simulink model "bandpass_complex_PAM_channel"  (R2016b)
settings: Solver=ode45  StartTime=0.0  StopTime=1000  RelTol=1e-3  EnableMultiTasking=on
InitFcn:
  | close all;
  | bandpass_complex_PAM_channel_ini;
StopFcn:
  | figure(1),
  | n=1:min([1000 length(srx)]);
  | subplot(211),plot(n,real(srx(n)),'.');
  | title('Real(srx)');
  | subplot(212),plot(n,imag(srx(n)),'.');
  | title('Imag(srx)');
undefined symbols (not defined in the file or in its folder): j
libraries: commfilt2 x2, commnoisgen2 x1, commrandsrc2 x1, commdigbbndam3 x1, commsink2 x1, commutil2 x1, dspobslib x1
settings Model: Creator=erban  LastModifiedBy=erban
settings DataIOCC: LimitDataPoints=on  SaveFormat=Array  SignalLoggingSaveFormat=ModelDataLogs  SignalLoggingName=sigsOut
settings OptimizationCC: BooleanDataType=off
settings DebuggingCC: SaveWithParameterizedLinksMsg=none  UnderspecifiedInitializationDetection=Classic  MergeDetectMultiDrivingBlocksExec=none  SignalResolutionControl=TryResolveAllWithWarning  MultiTaskDSMMsg=warning  MultiTaskCondExecSysMsg=none
settings HardwareCC: ProdBitPerPointer=32  ProdBitPerSizeT=32  ProdBitPerPtrDiffT=32  ProdLargestAtomicFloat=None  ProdIntDivRoundTo=Undefined  ProdEndianess=Unspecified  ProdWordSize=32  ProdHWDeviceType=32-bit Generic  TargetUnknown=on
settings ModelReferenceCC: PropagateSignalLabelsOutOfModel=off
settings GRTTargetCC: TargetLangStandard=C89/C90 (ANSI)  CombineOutputUpdateFcns=off  GRTInterface=on
settings ConfigComp: CovMetricSettings=dw  CovHtmlReporting=on  CovSaveCumulativeToWorkspaceVar=on  CovSaveSingleToWorkspaceVar=on  CovExternalEMLEnable=off

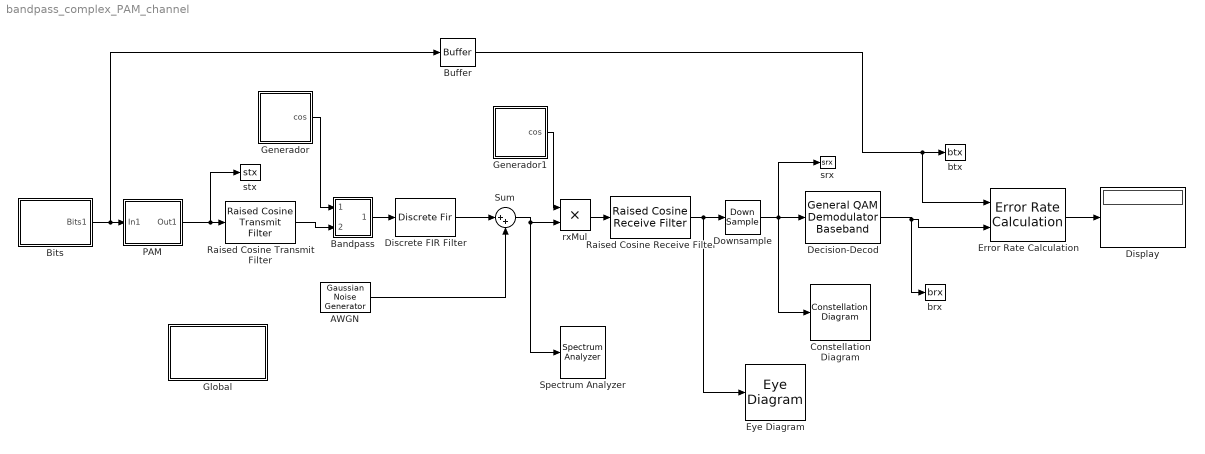
== system bandpass_complex_PAM_channel ==
  AWGN : commnoisgen2/Gaussian Noise Generator  m=0  d=1e-6  s=floor(60 * rand)+1  Ts=-1  frameBased=off  sampPerFrame=64  orient=off  outDataType=double
  Bandpass : Subsystem
      mask Display: disp('x Re{.}');
  Bits : Subsystem
      mask Display: disp('11001010');
  Buffer : Buffer  N=2  TreatMby1Signals=One channel  OutputFrames=off
  Constellation Diagram : ConstellationDiagram
  Decision-Decod : commdigbbndam3/General QAM Demodulator Baseband  SigCon=[1+j,-1+j,1-j,-1-j]  OutType=Bit  DecType=Hard decision  VarSource=Dialog  Variance=1  outDtypeBit=Inherit via internal rule  outDtype=Inherit via internal rule  roundingMode=Floor  overflowMode=Wrap  OvFlMode=off  OvFlModeLastStrValue=off  sigConstWordLen=16  sigConstDataTypeStr=Inherit: Same word length as input  sigConstLastDataTypeStr=Inherit: Same word length as input  accum1WordLen=32  accum1FracLen=30  prodInWordLen=32  prodInFracLen=30  prodInDataTypeStr=Inherit: Same as accumulator 1  prodInLastDataTypeStr=Inherit: Same as accumulator 1  prodOutWordLen=32  prodOutFracLen=30  accum2WordLen=32  accum2FracLen=30  accum3WordLen=32  accum3FracLen=30  nsiWordLen=32  nsiFracLen=30  nsiDataTypeStr=Inherit: Same as accumulator 3  nsiLastDataTypeStr=Inherit: Same as accumulator 3  invn0WordLen=16  invn0FracLen=8  invn0DataTypeStr=Inherit: Same word length as input  invn0LastDataTypeStr=Inherit: Same word length as input  outputWordLen=32  outputFracLen=30
  Discrete FIR Filter : DiscreteFir  Coefficients=1
  Display : Display
  Downsample : DownSample  N=128  RateOptions=Allow multirate processing
  Error Rate Calculation : commsink2/Error Rate Calculation  N=20  st_delay=50  cp_mode=Entire frame  subframe=[]  PMode=Port  WsName=ErrorVec  RsMode2=off  stop=off  numErr=100  maxBits=1e6
  Eye Diagram : EyeDiagram
  Generador : Subsystem  mask(SenCos){desfase=0, frec=1e4}
      mask prompts: frec "Frecuencia (Hz)"
      mask help: Saca un seno y un coseno de la frecuencia y la fase dadas.
      mask Display: disp('Complex \n exp(j.)');
  Generador1 : Subsystem  mask(SenCos){desfase=0, frec=10000}
      mask prompts: frec "Frecuencia (Hz)"
      mask help: Saca un seno y un coseno de la frecuencia y la fase dadas.
      mask Display: disp('Complex \n exp(-j.)');
  Global : Subsystem  mask{constellation=[1+j,-1+j,1-j,-1-j], Rb=1000, fc=1e4, NoiseVar=1e-6, channel=1, CFreqD=0, CPhasD=0, SPerD=0, SPhasD=0}
      mask prompts: fc "fc (Hz)"; channel "FIR channel"; CFreqD "Freq. Dev. (% fc)"; CPhasD "Phase Dev. (rad)"; SPerD "Symbol Period Dev. (% T)"; SPhasD "Symbol Phase Dev. (% T)"
      mask Display: disp('NoiseVar \n Constellation \n Rb \n ...')
  PAM : Subsystem  mask{cnstl=[1+j,-1+j,1-j,-1-j]}
      mask prompts: cnstl "Constelation"
      mask help: Codificador.
      mask Display: disp('Symbol \n Encoder');
  Raised Cosine Receive Filter : commfilt2/Raised Cosine Receive Filter  filtType=Square root  R=1  filtSpan=10  N=128  downFactor=1  downOffset=0  filterGain=1  InputProcessing=Columns as channels (frame based)  RateOptions=Allow multirate processing  framing=Mute  checkCoeff=off  variableName=rcRxFilt  currentFiltSpan=10  D=5  inputOffset=0  sampMode=Mute  saveAsFlag=0  rateMode=Downsampling  checkGain=Normalized  launchFVT=on  roundingMode=Floor  overflowMode=off  coeffDataTypeStr=Inherit: Same word length as input  coeffMin=[]  coeffMax=[]  coeffLastDataTypeStr=Inherit: Same word length as input  accumDataTypeStr=Inherit: Same as product output  accumLastDataTypeStr=Inherit: Same as product output  outputDataTypeStr=Inherit: Same as accumulator  outputMin=[]  outputMax=[]  outputLastDataTypeStr=Inherit: Same as accumulator
  Raised Cosine Transmit Filter : commfilt2/Raised Cosine Transmit Filter  filtType=Square root  R=1  filtSpan=10  N=128  filterGain=1  InputProcessing=Columns as channels (frame based)  RateOptions=Allow multirate processing  framing=Mute  checkCoeff=on  variableName=bbb  checkGain=Normalized  sampMode=Mute  saveAsFlag=0  currentFiltSpan=10  D=(10)/2  launchFVT=on  roundingMode=Floor  overflowMode=off  coeffDataTypeStr=Inherit: Same word length as input  coeffMin=[]  coeffMax=[]  coeffLastDataTypeStr=Inherit: Same word length as input  outputDataTypeStr=Inherit: Same as accumulator  outputMin=[]  outputMax=[]  outputLastDataTypeStr=Inherit: Same as accumulator
  Spectrum Analyzer : SpectrumAnalyzer
  Sum : Sum  Inputs=|++  SaturateOnIntegerOverflow=on
  brx : ToWorkspace  VariableName=brx  SampleTime=-1
      settings: Save2DSignal=2-D array (concatenate along first dimension)
  btx : ToWorkspace  VariableName=btx  SampleTime=-1
      settings: Save2DSignal=2-D array (concatenate along first dimension)
  rxMul : Product  Inputs=**
  srx : ToWorkspace  VariableName=srx  SampleTime=-1
      settings: Save2DSignal=2-D array (concatenate along first dimension)
  stx : ToWorkspace  VariableName=stx  SampleTime=-1
      settings: Save2DSignal=2-D array (concatenate along first dimension)
  wires:
  PAM/1(Out1) -> stx/1, Raised Cosine Transmit Filter/1
  AWGN/1 -> Sum/2
  Raised Cosine Receive Filter/1 -> Downsample/1, Eye Diagram/1
  Error Rate Calculation/1 -> Display/1
  Raised Cosine Transmit Filter/1 -> Bandpass/2(In2)
  Downsample/1 -> srx/1, Constellation Diagram/1, Decision-Decod/1
  Sum/1 -> Spectrum Analyzer/1, rxMul/2
  rxMul/1 -> Raised Cosine Receive Filter/1
  Generador1/1(cos) -> rxMul/1
  Generador/1(cos) -> Bandpass/1(In1)
  Bits/1(Bits1) -> PAM/1(In1), Buffer/1
  Decision-Decod/1 -> Error Rate Calculation/2, brx/1
  Buffer/1 -> Error Rate Calculation/1, btx/1
  Discrete FIR Filter/1 -> Sum/1
  Bandpass/1(Out1) -> Discrete FIR Filter/1

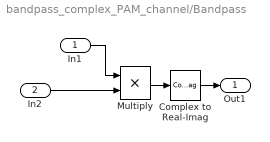
== system bandpass_complex_PAM_channel/Bandpass ==
  In1 : Inport
  In2 : Inport  Port=2
  Complex to Real-Imag : ComplexToRealImag  Output=Real
  Multiply : Product  Inputs=**
  Out1 : Outport
  wires:
  Multiply/1 -> Complex to Real-Imag/1
  In2/1 -> Multiply/2
  Complex to Real-Imag/1 -> Out1/1
  In1/1 -> Multiply/1

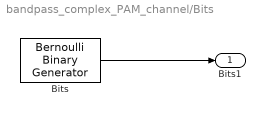
== system bandpass_complex_PAM_channel/Bits ==
  Bits : commrandsrc2/Bernoulli Binary Generator  P=0.5  seed=floor(60 * rand)+1  Ts=0.001  frameBased=off  sampPerFrame=1  orient=off  outDataType=double
  Bits1 : Outport
  wires:
  Bits/1 -> Bits1/1

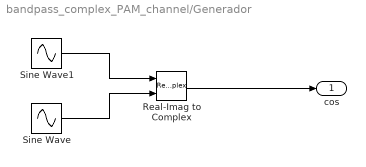
== system bandpass_complex_PAM_channel/Generador ==
  Real-Imag to Complex : RealImagToComplex
  Sine Wave : Sin  Amplitude=sqrt(2)  Frequency=2*pi*frec  Phase=desfase
  Sine Wave1 : Sin  Amplitude=sqrt(2)  Frequency=2*pi*frec  Phase=pi/2+desfase
  cos : Outport
  wires:
  Sine Wave/1 -> Real-Imag to Complex/2
  Real-Imag to Complex/1 -> cos/1
  Sine Wave1/1 -> Real-Imag to Complex/1

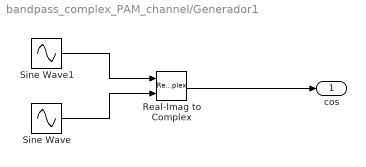
== system bandpass_complex_PAM_channel/Generador1 ==
  Real-Imag to Complex : RealImagToComplex
  Sine Wave : Sin  Amplitude=-sqrt(2)  Frequency=2*pi*frec  Phase=desfase
  Sine Wave1 : Sin  Amplitude=sqrt(2)  Frequency=2*pi*frec  Phase=pi/2+desfase
  cos : Outport
  wires:
  Sine Wave/1 -> Real-Imag to Complex/2
  Real-Imag to Complex/1 -> cos/1
  Sine Wave1/1 -> Real-Imag to Complex/1

== system bandpass_complex_PAM_channel/Global ==

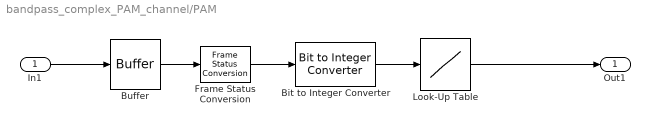
== system bandpass_complex_PAM_channel/PAM ==
  In1 : Inport
  Bit to Integer Converter : commutil2/Bit to Integer Converter  nbits=log2(length(cnstl))  bitOrder=MSB first  signedOutputValues=Unsigned  outDtype=Inherit via internal rule  outDtypeSigned=Inherit via internal rule
  Buffer : Buffer  N=log2(length(cnstl))  TreatMby1Signals=One channel
  Frame Status Conversion : dspobslib/Frame Status Conversion  growRefPort=off  outframe=Sample-based
  Look-Up Table : Lookup  InputValues=[0:length(cnstl)-1]  Table=cnstl  SaturateOnIntegerOverflow=on
  Out1 : Outport
  wires:
  Frame Status Conversion/1 -> Bit to Integer Converter/1
  In1/1 -> Buffer/1
  Buffer/1 -> Frame Status Conversion/1
  Look-Up Table/1 -> Out1/1
  Bit to Integer Converter/1 -> Look-Up Table/1
